simulink model "aerodynamic_tests"  (R2020a)
settings: Solver=FixedStepAuto  StartTime=0.0  StopTime=5  FixedStep=1e-5  RelTol=1e-3
undefined symbols (not defined in the file or in its folder): A4, AQ3483, AS4, BB3483
libraries: simulink x2, aerolibconvert2 x1
settings Model: SimulationMode=accelerator  Creator=rag  LastModifiedBy=rag

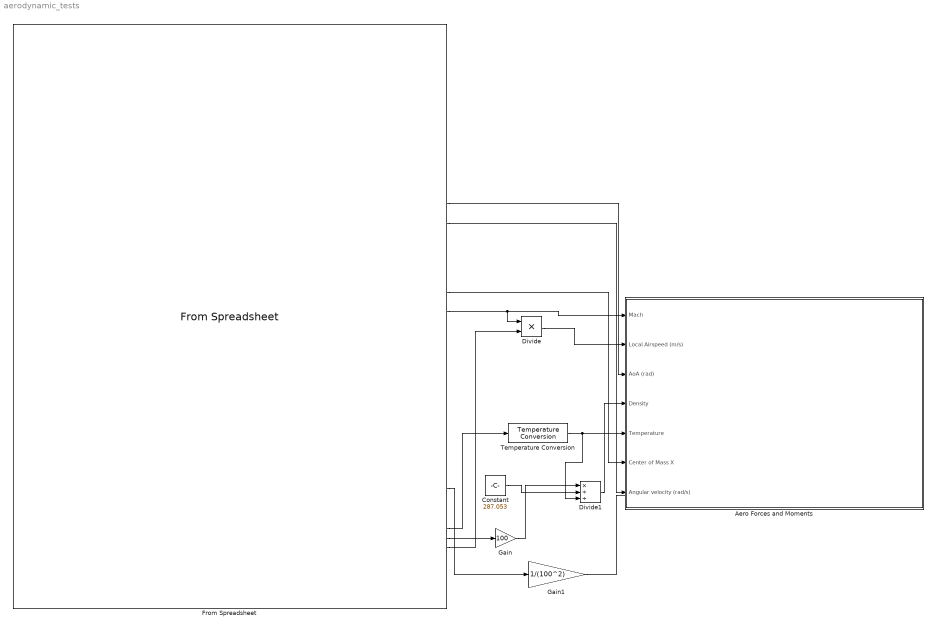
== system aerodynamic_tests ==
  Aero Forces and Moments : Subsystem
  Constant : Constant  Value=287.053
  Divide : Product  Inputs=**
  Divide1 : Product  Inputs=*//
  From Spreadsheet : FromSpreadsheet  FileName=C:\Users\rag\Documents\GitHub\EPQ\OpenRocket\full simulation F15 east 2.xlsx  SheetName=full simulation F15 east 2  Range=A4:AQ3483,AS4:BB3483  ExtrapolationBeforeFirstDataPoint=Hold first value  InterpolationWithinTimeRange=Zero order hold  ExtrapolationAfterLastDataPoint=Hold last value
  Gain : Gain  Gain=100
  Gain1 : Gain  Gain=1/(100^2)
  Temperature Conversion : aerolibconvert2/Temperature Conversion  IU=C  OU=K
      settings: SourceProductBaseCode=AE
  wires:
  From Spreadsheet/26 -> Divide/1, Aero Forces and Moments/1(Mach)
  From Spreadsheet/15 -> Aero Forces and Moments/3(AoA (rad))
  Divide1/1 -> Aero Forces and Moments/4(Density)
  From Spreadsheet/24 -> Aero Forces and Moments/6(Center of Mass X)
  From Spreadsheet/17 -> Aero Forces and Moments/7(Angular velocity (rad/s))
  Divide/1 -> Aero Forces and Moments/2(Local Airspeed (m/s))
  Temperature Conversion/1 -> Divide1/3, Aero Forces and Moments/5(Temperature)
  From Spreadsheet/48 -> Temperature Conversion/1
  From Spreadsheet/50 -> Divide/2
  Constant/1 -> Divide1/2
  From Spreadsheet/49 -> Gain/1
  Gain/1 -> Divide1/1
  Gain1/1 -> ?
  From Spreadsheet/44 -> Gain1/1

== system aerodynamic_tests/Aero Forces and Moments ==
  Mach : Inport
  Local Airspeed (m/s) : Inport  Port=2
  AoA (rad) : Inport  Port=3
  Density : Inport  Port=4
  Temperature : Inport  Port=5
  Center of Mass X : Inport  Port=6
  Angular velocity (rad/s) : Inport  Port=7
  Axial Drag Calculator : Subsystem
  CN and Cm calculator : Subsystem
  Constants : Subsystem
  wires:
  AoA (rad)/1 -> Axial Drag Calculator/2(AoA (rad)), CN and Cm calculator/3(AoA (rads))
  Temperature/1 -> Axial Drag Calculator/4(Temperature)
  Mach/1 -> CN and Cm calculator/1(Mach), Axial Drag Calculator/1(Mach)
  Density/1 -> Axial Drag Calculator/3(Density)
  Angular velocity (rad/s)/1 -> CN and Cm calculator/5(Angular Velocity (rad/s))
  Center of Mass X/1 -> CN and Cm calculator/4(Center of Mass X)
  Local Airspeed (m/s)/1 -> Axial Drag Calculator/13(Airspeed), CN and Cm calculator/2(Airspeed (m/s))
  Constants/1(Reference diameter (m)) -> CN and Cm calculator/7(Reference Diameter (m))
  Constants/3(Reference area (m^2)) -> Axial Drag Calculator/9(Reference Area (m^2)), CN and Cm calculator/8(Reference Area (m^2))
  Constants/4(Nose Cone Length (m)) -> Axial Drag Calculator/10(Nose Cone Length (m)), CN and Cm calculator/9(Nose Cone Length (m))
  Constants/5(Body Tube Length (m)) -> Axial Drag Calculator/5(Body Tube Length (m)), CN and Cm calculator/10(Body Tube Length (m))
  Constants/8(Nose Cone Planform Area (m^2)) -> CN and Cm calculator/11(Nose Cone Planform Area (m^2))
  Constants/9(Body Tube Planform Area (m^2)) -> CN and Cm calculator/12(Body Tube Planform Area (m^2))
  Constants/12(Body Tube CP (m)) -> CN and Cm calculator/13(Body Tube CP)
  Constants/13(Nose Cone CP (m)) -> CN and Cm calculator/14(Nose Cone CP)
  Constants/14(Pitch Center X (m)) -> CN and Cm calculator/15(Pitch Center X)
  Constants/7(Body Tube Wet Area (m^2)) -> Axial Drag Calculator/6(Body Tube Wet Area (m^2))
  Constants/6("Nose Cone Wet Area (m^2) ") -> Axial Drag Calculator/7(Nose Cone Wet Area (m^2))
  Constants/2(Reference radius (m)) -> Axial Drag Calculator/8(Reference Radius (m))
  Constants/10(Surface Roughness (m)) -> Axial Drag Calculator/11(Surface Roughness)
  Constants/11(sin(phi)) -> Axial Drag Calculator/12(sinphi)

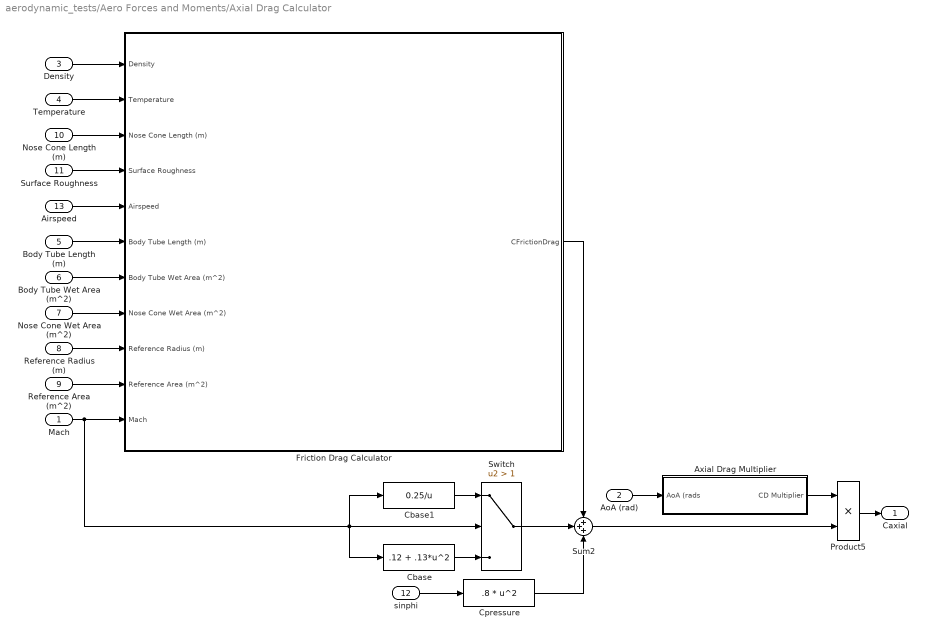
== system aerodynamic_tests/Aero Forces and Moments/Axial Drag Calculator ==
  Mach : Inport
  AoA (rad) : Inport  Port=2
  Density : Inport  Port=3
  Temperature : Inport  Port=4
  Body Tube Length (m) : Inport  Port=5
  Body Tube Wet Area (m^2) : Inport  Port=6
  Nose Cone Wet Area (m^2) : Inport  Port=7
  Reference Radius (m) : Inport  Port=8
  Reference Area (m^2) : Inport  Port=9
  Nose Cone Length (m) : Inport  Port=10
  Surface Roughness : Inport  Port=11
  sinphi : Inport  Port=12
  Airspeed : Inport  Port=13
  Axial Drag Multiplier : Subsystem
  Cbase : Fcn  Expr=.12 + .13*u^2
  Cbase1 : Fcn  Expr=0.25/u
  Cpressure : Fcn  Expr=.8 * u^2
  Friction Drag Calculator : Subsystem
  Product5 : Product
  Sum2 : Sum  Inputs=+++
  Switch : Switch  Criteria=u2 > Threshold  Threshold=1
  Caxial : Outport  VectorParamsAs1DForOutWhenUnconnected=off
  wires:
  Nose Cone Wet Area (m^2)/1 -> Friction Drag Calculator/8(Nose Cone Wet Area (m^2))
  Reference Area (m^2)/1 -> Friction Drag Calculator/10(Reference Area (m^2))
  Reference Radius (m)/1 -> Friction Drag Calculator/9(Reference Radius (m))
  Body Tube Wet Area (m^2)/1 -> Friction Drag Calculator/7(Body Tube Wet Area (m^2))
  sinphi/1 -> Cpressure/1
  Airspeed/1 -> Friction Drag Calculator/5(Airspeed)
  Surface Roughness/1 -> Friction Drag Calculator/4(Surface Roughness)
  Temperature/1 -> Friction Drag Calculator/2(Temperature)
  Mach/1 -> Cbase/1, Cbase1/1, Switch/2, Friction Drag Calculator/11(Mach)
  Density/1 -> Friction Drag Calculator/1(Density)
  Nose Cone Length (m)/1 -> Friction Drag Calculator/3(Nose Cone Length (m))
  Body Tube Length (m)/1 -> Friction Drag Calculator/6(Body Tube Length (m))
  Product5/1 -> Caxial/1
  Friction Drag Calculator/1(CFrictionDrag) -> Sum2/1
  Cbase/1 -> Switch/3
  Cpressure/1 -> Sum2/3
  AoA (rad)/1 -> Axial Drag Multiplier/1(AoA (rads)
  Sum2/1 -> Product5/2
  Axial Drag Multiplier/1(CD Multiplier) -> Product5/1
  Cbase1/1 -> Switch/1
  Switch/1 -> Sum2/2

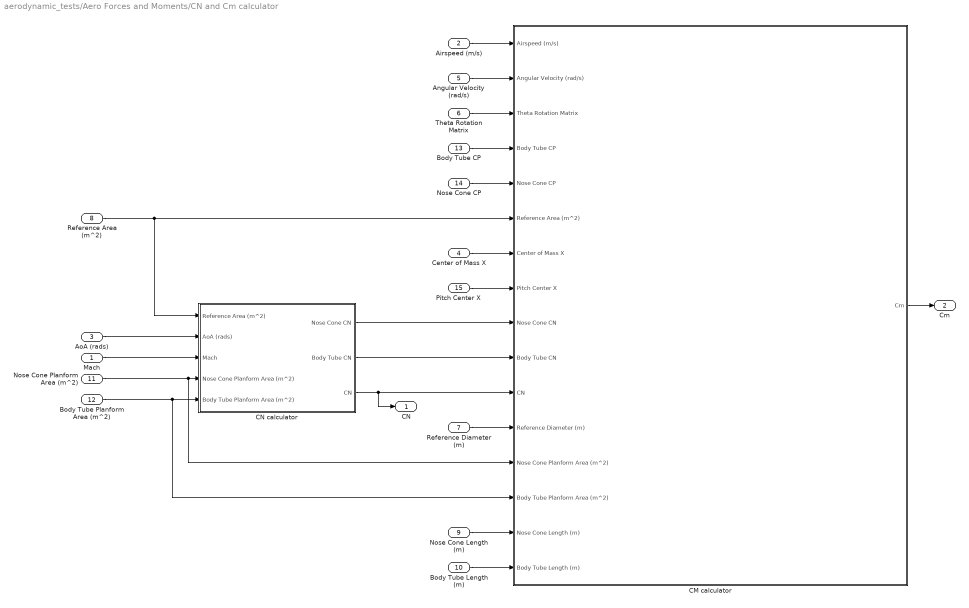
== system aerodynamic_tests/Aero Forces and Moments/CN and Cm calculator ==
  Mach : Inport
  Airspeed (m/s) : Inport  Port=2
  AoA (rads) : Inport  Port=3
  Center of Mass X : Inport  Port=4
  Angular Velocity (rad/s) : Inport  Port=5
  Theta Rotation Matrix : Inport  Port=6
  Reference Diameter (m) : Inport  Port=7
  Reference Area (m^2) : Inport  Port=8
  Nose Cone Length (m) : Inport  Port=9
  Body Tube Length (m) : Inport  Port=10
  Nose Cone Planform Area (m^2) : Inport  Port=11
  Body Tube Planform Area (m^2) : Inport  Port=12
  Body Tube CP : Inport  Port=13
  Nose Cone CP : Inport  Port=14
  Pitch Center X : Inport  Port=15
  CM calculator : Subsystem
  CN calculator : Subsystem
  CN : Outport  VectorParamsAs1DForOutWhenUnconnected=off
  Cm : Outport  Port=2  VectorParamsAs1DForOutWhenUnconnected=off
  wires:
  Body Tube Planform Area (m^2)/1 -> CM calculator/14(Body Tube Planform Area (m^2)), CN calculator/5(Body Tube Planform Area (m^2))
  Pitch Center X/1 -> CM calculator/8(Pitch Center X)
  Nose Cone CP/1 -> CM calculator/5(Nose Cone CP)
  Body Tube CP/1 -> CM calculator/4(Body Tube CP)
  Nose Cone Planform Area (m^2)/1 -> CM calculator/13(Nose Cone Planform Area (m^2)), CN calculator/4(Nose Cone Planform Area (m^2))
  Angular Velocity (rad/s)/1 -> CM calculator/2(Angular Velocity (rad/s))
  Reference Area (m^2)/1 -> CN calculator/1(Reference Area (m^2)), CM calculator/6(Reference Area (m^2))
  AoA (rads)/1 -> CN calculator/2(AoA (rads))
  Mach/1 -> CN calculator/3(Mach)
  Center of Mass X/1 -> CM calculator/7(Center of Mass X)
  CN calculator/3(CN) -> CN/1, CM calculator/11(CN)
  CN calculator/2(Body Tube CN) -> CM calculator/10(Body Tube CN)
  CN calculator/1(Nose Cone CN) -> CM calculator/9(Nose Cone CN)
  Airspeed (m/s)/1 -> CM calculator/1(Airspeed (m/s))
  Theta Rotation Matrix/1 -> CM calculator/3(Theta Rotation Matrix)
  Reference Diameter (m)/1 -> CM calculator/12(Reference Diameter (m))
  Nose Cone Length (m)/1 -> CM calculator/15(Nose Cone Length (m))
  CM calculator/1(Cm) -> Cm/1
  Body Tube Length (m)/1 -> CM calculator/16(Body Tube Length (m))

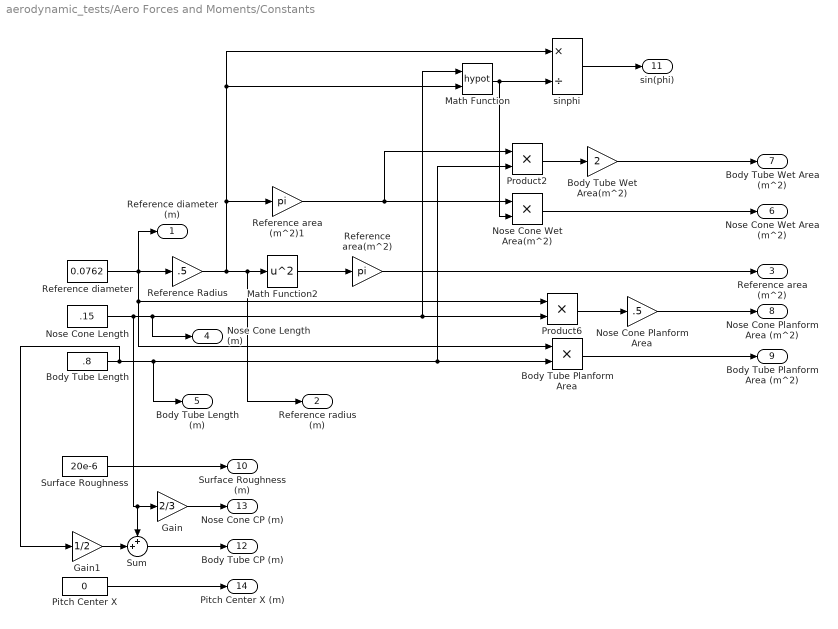
== system aerodynamic_tests/Aero Forces and Moments/Constants ==
  Body Tube Length : Constant  Value=.8
  Body Tube Planform Area : Product
  Body Tube Wet Area(m^2) : Gain  Gain=2
  Gain : Gain  Gain=2/3
  Gain1 : Gain  Gain=1/2
  Math Function : Math  Operator=hypot  SignedPower=on  SaturateOnIntegerOverflow=on
  Math Function2 : Math  Operator=square  SignedPower=on  SaturateOnIntegerOverflow=on
  Nose Cone Length : Constant  Value=.15
  Nose Cone Planform Area : Gain  Gain=.5
  Nose Cone Wet Area(m^2) : Product
  Pitch Center X : Constant  Value=0
  Product2 : Product
  Product6 : Product
  Reference Radius : Gain  Gain=.5
  Reference area (m^2)1 : Gain  Gain=pi
  Reference area(m^2) : Gain  Gain=pi
  Reference diameter : Constant  Value=0.0762
  Sum : Sum  Inputs=++|
  Surface Roughness : Constant  Value=20e-6
  sinphi : Product  Inputs=*/
  Reference diameter (m) : Outport  VectorParamsAs1DForOutWhenUnconnected=off
  Reference radius (m) : Outport  Port=2  VectorParamsAs1DForOutWhenUnconnected=off
  Reference area (m^2) : Outport  Port=3  VectorParamsAs1DForOutWhenUnconnected=off
  Nose Cone Length (m) : Outport  Port=4  VectorParamsAs1DForOutWhenUnconnected=off
  Body Tube Length (m) : Outport  Port=5  VectorParamsAs1DForOutWhenUnconnected=off
  "Nose Cone Wet Area (m^2) " : Outport  Port=6  VectorParamsAs1DForOutWhenUnconnected=off
  Body Tube Wet Area (m^2) : Outport  Port=7  VectorParamsAs1DForOutWhenUnconnected=off
  Nose Cone Planform Area (m^2) : Outport  Port=8  VectorParamsAs1DForOutWhenUnconnected=off
  Body Tube Planform Area (m^2) : Outport  Port=9  VectorParamsAs1DForOutWhenUnconnected=off
  Surface Roughness (m) : Outport  Port=10  VectorParamsAs1DForOutWhenUnconnected=off
  sin(phi) : Outport  Port=11  VectorParamsAs1DForOutWhenUnconnected=off
  Body Tube CP (m) : Outport  Port=12  VectorParamsAs1DForOutWhenUnconnected=off
  Nose Cone CP (m) : Outport  Port=13  VectorParamsAs1DForOutWhenUnconnected=off
  Pitch Center X (m) : Outport  Port=14  VectorParamsAs1DForOutWhenUnconnected=off
  wires:
  Reference diameter/1 -> Reference diameter (m)/1, Body Tube Planform Area/1, Product6/1, Reference Radius/1
  Math Function2/1 -> Reference area(m^2)/1
  Nose Cone Length/1 -> Product6/2, Math Function/1, Nose Cone Length (m)/1, Sum/1, Gain/1
  Product6/1 -> Nose Cone Planform Area/1
  Reference Radius/1 -> Math Function2/1, Reference radius (m)/1, Math Function/2, sinphi/1, Reference area (m^2)1/1
  Reference area (m^2)1/1 -> Product2/1, Nose Cone Wet Area(m^2)/1
  Product2/1 -> Body Tube Wet Area(m^2)/1
  Math Function/1 -> Nose Cone Wet Area(m^2)/2, sinphi/2
  Reference area(m^2)/1 -> Reference area (m^2)/1
  Nose Cone Wet Area(m^2)/1 -> "Nose Cone Wet Area (m^2) "/1
  Body Tube Wet Area(m^2)/1 -> Body Tube Wet Area (m^2)/1
  Body Tube Planform Area/1 -> Body Tube Planform Area (m^2)/1
  Nose Cone Planform Area/1 -> Nose Cone Planform Area (m^2)/1
  Surface Roughness/1 -> Surface Roughness (m)/1
  sinphi/1 -> sin(phi)/1
  Sum/1 -> Body Tube CP (m)/1
  Gain/1 -> Nose Cone CP (m)/1
  Pitch Center X/1 -> Pitch Center X (m)/1
  Gain1/1 -> Sum/2
  Body Tube Length/1 -> Gain1/1, Body Tube Length (m)/1, Body Tube Planform Area/2, Product2/2

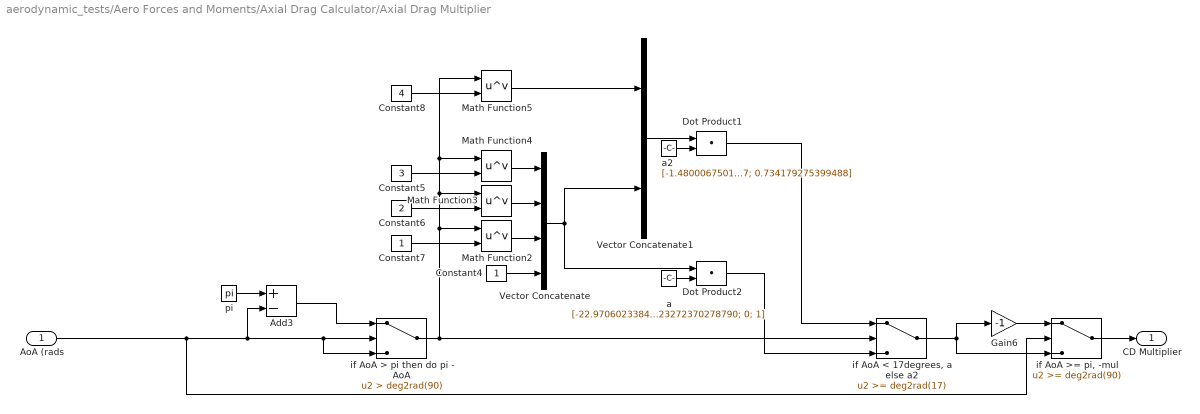
== system aerodynamic_tests/Aero Forces and Moments/Axial Drag Calculator/Axial Drag Multiplier ==
  AoA (rads : Inport
  Add3 : Sum  Inputs=+-
  Constant4 : Constant
  Constant5 : Constant  Value=3
  Constant6 : Constant  Value=2
  Constant7 : Constant
  Constant8 : Constant  Value=4
  Dot Product1 : DotProduct  SaturateOnIntegerOverflow=on  OutDataTypeStr=Inherit: Inherit via internal rule
  Dot Product2 : DotProduct  SaturateOnIntegerOverflow=on  OutDataTypeStr=Inherit: Inherit via internal rule
  Gain6 : Gain  Gain=-1
  Math Function{2..5} (4 alike) : Math  Operator=pow  SignedPower=on  SaturateOnIntegerOverflow=on
  Vector Concatenate : Concatenate  NumInputs=4
  Vector Concatenate1 : Concatenate
  a : Constant  Value=[-22.970602338418825; 10.223272370278790; 0; 1]
  a2 : Constant  Value=[-1.480006750190687; 6.784940235048046; -10.062655893223173; 4.334008218595027; 0.734179275399488]
  "if AoA < 17degrees, a else a2" : Switch  Threshold=deg2rad(17)
  if AoA > pi then do pi - AoA : Switch  Criteria=u2 > Threshold  Threshold=deg2rad(90)
  "if AoA >= pi, -mul" : Switch  Threshold=deg2rad(90)
  pi : Constant  Value=pi
  CD Multiplier : Outport  VectorParamsAs1DForOutWhenUnconnected=off
  wires:
  Constant4/1 -> Vector Concatenate/4
  Constant5/1 -> Math Function4/2
  if AoA > pi then do pi - AoA/1 -> Math Function5/1, Math Function4/1, Math Function3/1, Math Function2/1, "if AoA < 17degrees, a else a2"/2
  Add3/1 -> if AoA > pi then do pi - AoA/1
  Vector Concatenate1/1 -> Dot Product1/1
  AoA (rads/1 -> "if AoA >= pi, -mul"/2, Add3/2, if AoA > pi then do pi - AoA/3, if AoA > pi then do pi - AoA/2
  a/1 -> Dot Product2/2
  "if AoA >= pi, -mul"/1 -> CD Multiplier/1
  Math Function4/1 -> Vector Concatenate/1
  "if AoA < 17degrees, a else a2"/1 -> "if AoA >= pi, -mul"/3, Gain6/1
  Gain6/1 -> "if AoA >= pi, -mul"/1
  pi/1 -> Add3/1
  Constant7/1 -> Math Function2/2
  Vector Concatenate/1 -> Vector Concatenate1/2, Dot Product2/1
  Math Function2/1 -> Vector Concatenate/3
  Constant6/1 -> Math Function3/2
  Dot Product2/1 -> "if AoA < 17degrees, a else a2"/3
  Constant8/1 -> Math Function5/2
  a2/1 -> Dot Product1/2
  Math Function5/1 -> Vector Concatenate1/1
  Math Function3/1 -> Vector Concatenate/2
  Dot Product1/1 -> "if AoA < 17degrees, a else a2"/1

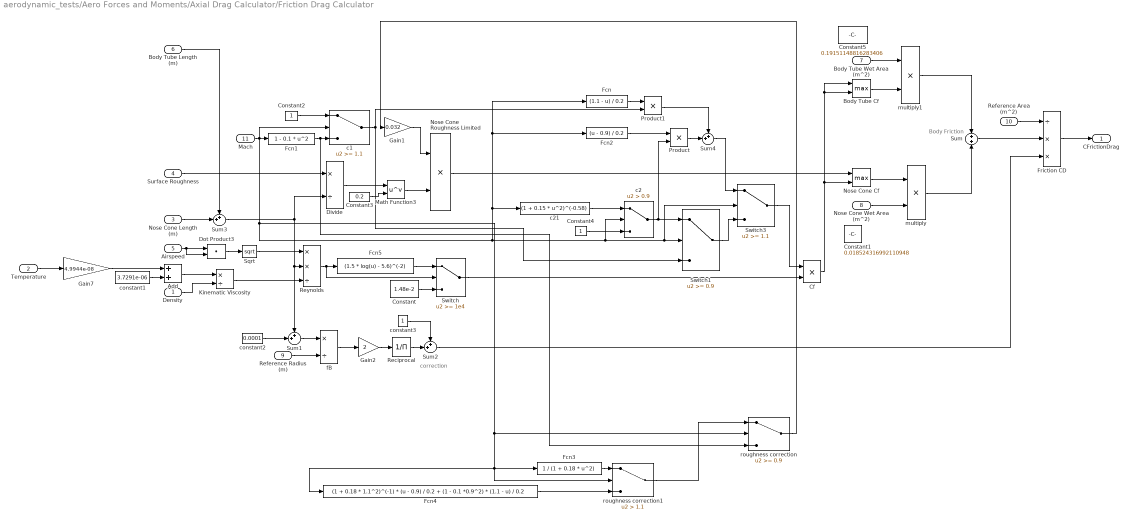
== system aerodynamic_tests/Aero Forces and Moments/Axial Drag Calculator/Friction Drag Calculator ==
  note: correction
  note: Body Friction
  Density : Inport
  Temperature : Inport  Port=2
  Nose Cone Length (m) : Inport  Port=3
  Surface Roughness : Inport  Port=4
  Airspeed : Inport  Port=5
  Body Tube Length (m) : Inport  Port=6
  Body Tube Wet Area (m^2) : Inport  Port=7
  Nose Cone Wet Area (m^2) : Inport  Port=8
  Reference Radius (m) : Inport  Port=9
  Reference Area (m^2) : Inport  Port=10
  Mach : Inport  Port=11
  Add : Sum
  Body Tube Cf : MinMax  Function=max  Inputs=2
  Cf : Product  Inputs=**
  Constant : Constant  Value=1.48e-2
  Constant1 : Constant  Value=0.018524316992110948
  Constant2 : Constant
  Constant3 : Constant  Value=0.2
  Constant4 : Constant
  Constant5 : Constant  Value=0.19151148816283406
  Divide : Product  Inputs=*/
  Dot Product3 : DotProduct  SaturateOnIntegerOverflow=on  OutDataTypeStr=Inherit: Inherit via internal rule
  Fcn : Fcn  Expr=(1.1 - u) / 0.2
  Fcn1 : Fcn  Expr=1 - 0.1 * u^2
  Fcn2 : Fcn  Expr=(u - 0.9) / 0.2
  Fcn3 : Fcn  Expr=1 / (1 + 0.18 * u^2)
  Fcn4 : Fcn  Expr=(1 + 0.18 * 1.1^2)^(-1) * (u - 0.9) / 0.2 + (1 - 0.1 *0.9^2) * (1.1 - u) / 0.2
  Fcn5 : Fcn  Expr=(1.5 * log(u) - 5.6)^(-2)
  Friction CD : Product  Inputs=/**
  Gain1 : Gain  Gain=0.032
  Gain2 : Gain  Gain=2
  Gain7 : Gain  Gain=4.9944e-08
  Kinematic Viscosity : Product  Inputs=*/
  Math Function3 : Math  Operator=pow  SignedPower=on  SaturateOnIntegerOverflow=on
  Nose Cone Cf : MinMax  Function=max  Inputs=2
  Nose Cone Roughness Limited : Product  Inputs=**
  Product : Product
  Product1 : Product
  Reciprocal : Product  Inputs=/
  Reynolds : Product  Inputs=**/
  Sqrt : Sqrt  SaturateOnIntegerOverflow=on
  Sum : Sum
  Sum{1..4} (4 alike) : Sum  Inputs=++|
  Switch : Switch  Threshold=1e4
  Switch1 : Switch  Threshold=0.9
  Switch3 : Switch  Threshold=1.1
  c1 : Switch  Threshold=1.1
  c2 : Switch  Criteria=u2 > Threshold  Threshold=0.9
  c21 : Fcn  Expr=(1 + 0.15 * u^2)^(-0.58)
  constant1 : Constant  Value=3.7291e-06
  constant2 : Constant  Value=0.0001
  constant3 : Constant
  fB : Product  Inputs=*/
  multiply : Product  Inputs=**
  multiply1 : Product  Inputs=**
  roughness correction : Switch  Threshold=0.9
  roughness correction1 : Switch  Criteria=u2 > Threshold  Threshold=1.1
  CFrictionDrag : Outport  VectorParamsAs1DForOutWhenUnconnected=off
  wires:
  Sqrt/1 -> Reynolds/1
  Kinematic Viscosity/1 -> Reynolds/3
  Constant3/1 -> Math Function3/2
  constant1/1 -> Add/2
  Add/1 -> Kinematic Viscosity/1
  Gain7/1 -> Add/1
  Reynolds/1 -> Switch/2, Fcn5/1
  Gain1/1 -> Nose Cone Roughness Limited/1
  Divide/1 -> Math Function3/1
  Math Function3/1 -> Nose Cone Roughness Limited/2
  Surface Roughness/1 -> Divide/1
  Temperature/1 -> Gain7/1
  Density/1 -> Kinematic Viscosity/2
  Nose Cone Roughness Limited/1 -> Nose Cone Cf/1
  Nose Cone Length (m)/1 -> Sum3/2
  Body Tube Length (m)/1 -> Sum3/1
  Cf/1 -> Body Tube Cf/1, Body Tube Cf/2, Nose Cone Cf/2
  Nose Cone Cf/1 -> multiply/1
  Nose Cone Wet Area (m^2)/1 -> multiply/2
  Body Tube Wet Area (m^2)/1 -> multiply1/1
  Body Tube Cf/1 -> multiply1/2
  multiply/1 -> Sum/2
  multiply1/1 -> Sum/1
  constant2/1 -> Sum1/2
  Sum1/1 -> fB/1
  Reference Radius (m)/1 -> fB/2
  fB/1 -> Gain2/1
  Gain2/1 -> Reciprocal/1
  Reciprocal/1 -> Sum2/2
  constant3/1 -> Sum2/1
  Sum/1 -> Friction CD/2
  Sum2/1 -> Friction CD/3
  Reference Area (m^2)/1 -> Friction CD/1
  Friction CD/1 -> CFrictionDrag/1
  Airspeed/1 -> Dot Product3/2, Dot Product3/1
  Dot Product3/1 -> Sqrt/1
  Switch/1 -> Cf/2
  Fcn5/1 -> Switch/1
  Constant/1 -> Switch/3
  c1/1 -> Product1/2, Switch1/3
  Fcn1/1 -> roughness correction/3, c1/3
  Constant2/1 -> c1/1
  c2/1 -> Product/2, Switch1/1
  Constant4/1 -> c2/3
  c21/1 -> c2/1
  Switch3/1 -> Cf/1
  Switch1/1 -> Switch3/3
  Fcn2/1 -> Product/1
  Product/1 -> Sum4/2
  Product1/1 -> Sum4/1
  Fcn/1 -> Product1/1
  Sum4/1 -> Switch3/1
  Fcn3/1 -> roughness correction1/1
  Mach/1 -> roughness correction/2, Fcn4/1, roughness correction1/2, Fcn3/1, Fcn/1, Fcn2/1, c21/1, c2/2, Switch3/2, Switch1/2, c1/2, Fcn1/1
  Fcn4/1 -> roughness correction1/3
  roughness correction1/1 -> roughness correction/1
  roughness correction/1 -> Gain1/1
  Sum3/1 -> Divide/2, Sum1/1, Reynolds/2

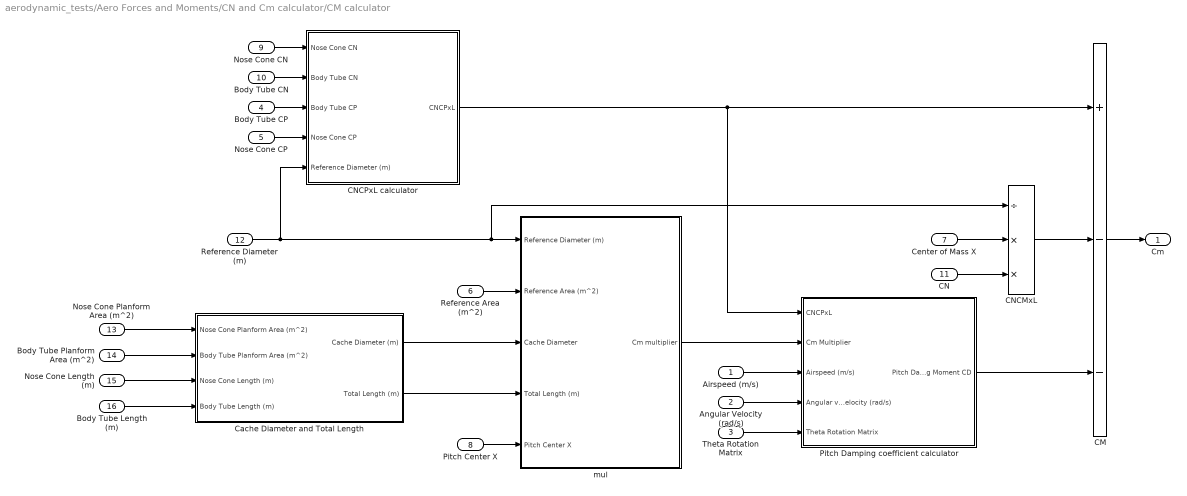
== system aerodynamic_tests/Aero Forces and Moments/CN and Cm calculator/CM calculator ==
  Airspeed (m/s) : Inport
  Angular Velocity (rad/s) : Inport  Port=2
  Theta Rotation Matrix : Inport  Port=3
  Body Tube CP : Inport  Port=4
  Nose Cone CP : Inport  Port=5
  Reference Area (m^2) : Inport  Port=6
  Center of Mass X : Inport  Port=7
  Pitch Center X : Inport  Port=8
  Nose Cone CN : Inport  Port=9
  Body Tube CN : Inport  Port=10
  CN : Inport  Port=11
  Reference Diameter (m) : Inport  Port=12
  Nose Cone Planform Area (m^2) : Inport  Port=13
  Body Tube Planform Area (m^2) : Inport  Port=14
  Nose Cone Length (m) : Inport  Port=15
  Body Tube Length (m) : Inport  Port=16
  CM : Sum  Inputs=+--
  CNCMxL : Product  Inputs=/**
  CNCPxL calculator : Subsystem
  Cache Diameter and Total Length : Subsystem
  Pitch Damping coefficient calculator : Subsystem
  mul : Subsystem
  Cm : Outport  VectorParamsAs1DForOutWhenUnconnected=off
  wires:
  CNCPxL calculator/1("CNCPxL ") -> Pitch Damping coefficient calculator/1(CNCPxL), CM/1
  Pitch Center X/1 -> mul/5(Pitch Center X)
  Cache Diameter and Total Length/2(Total Length (m)) -> mul/4(Total Length (m))
  Reference Diameter (m)/1 -> CNCMxL/1, mul/1(Reference Diameter (m)), CNCPxL calculator/5(Reference Diameter (m))
  Nose Cone CP/1 -> CNCPxL calculator/4(Nose Cone CP)
  CM/1 -> Cm/1
  Body Tube CP/1 -> CNCPxL calculator/3(Body Tube CP)
  Cache Diameter and Total Length/1(Cache Diameter (m)) -> mul/3(Cache Diameter)
  mul/1(Cm multiplier) -> Pitch Damping coefficient calculator/2(Cm Multiplier)
  Angular Velocity (rad/s)/1 -> Pitch Damping coefficient calculator/4(Angular velocity (rad/s))
  Airspeed (m/s)/1 -> Pitch Damping coefficient calculator/3(Airspeed (m/s))
  Reference Area (m^2)/1 -> mul/2(Reference Area (m^2))
  Theta Rotation Matrix/1 -> Pitch Damping coefficient calculator/5(Theta Rotation Matrix)
  Body Tube CN/1 -> CNCPxL calculator/2(Body Tube CN)
  Nose Cone CN/1 -> CNCPxL calculator/1(Nose Cone CN)
  Nose Cone Planform Area (m^2)/1 -> Cache Diameter and Total Length/1(Nose Cone Planform Area (m^2))
  Body Tube Planform Area (m^2)/1 -> Cache Diameter and Total Length/2(Body Tube Planform Area (m^2))
  Nose Cone Length (m)/1 -> Cache Diameter and Total Length/3(Nose Cone Length (m))
  Body Tube Length (m)/1 -> Cache Diameter and Total Length/4(Body Tube Length (m))
  Center of Mass X/1 -> CNCMxL/2
  CN/1 -> CNCMxL/3
  Pitch Damping coefficient calculator/1(Pitch Damping Moment CD) -> CM/3
  CNCMxL/1 -> CM/2

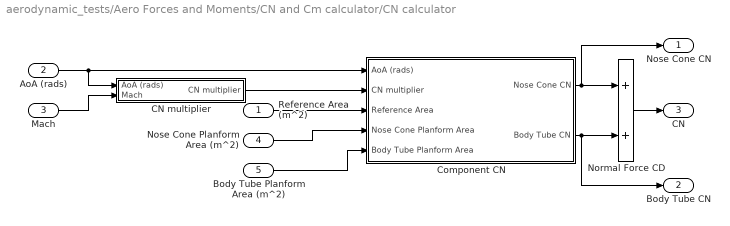
== system aerodynamic_tests/Aero Forces and Moments/CN and Cm calculator/CN calculator ==
  Reference Area (m^2) : Inport
  AoA (rads) : Inport  Port=2
  Mach : Inport  Port=3
  Nose Cone Planform Area (m^2) : Inport  Port=4
  Body Tube Planform Area (m^2) : Inport  Port=5
  CN multiplier : Subsystem
  Component CN : Subsystem
  Normal Force CD : Sum
  Nose Cone CN : Outport  VectorParamsAs1DForOutWhenUnconnected=off
  Body Tube CN : Outport  Port=2  VectorParamsAs1DForOutWhenUnconnected=off
  CN : Outport  Port=3  VectorParamsAs1DForOutWhenUnconnected=off
  wires:
  Mach/1 -> CN multiplier/2(Mach)
  CN multiplier/1(CN multiplier) -> Component CN/2(CN multiplier)
  Component CN/1(Nose Cone CN) -> Normal Force CD/1, Nose Cone CN/1
  AoA (rads)/1 -> CN multiplier/1(AoA (rads)), Component CN/1(AoA (rads))
  Nose Cone Planform Area (m^2)/1 -> Component CN/4(Nose Cone Planform Area)
  Component CN/2(Body Tube CN) -> Normal Force CD/2, Body Tube CN/1
  Body Tube Planform Area (m^2)/1 -> Component CN/5(Body Tube Planform Area)
  Reference Area (m^2)/1 -> Component CN/3(Reference Area)
  Normal Force CD/1 -> CN/1

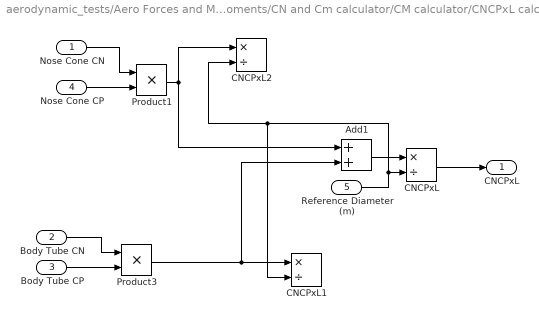
== system aerodynamic_tests/Aero Forces and Moments/CN and Cm calculator/CM calculator/CNCPxL calculator ==
  Nose Cone CN : Inport
  Body Tube CN : Inport  Port=2
  Body Tube CP : Inport  Port=3
  Nose Cone CP : Inport  Port=4
  Reference Diameter (m) : Inport  Port=5
  Add1 : Sum
  CNCPxL : Product  Inputs=*/
  CNCPxL1 : Product  Inputs=*/
  CNCPxL2 : Product  Inputs=*/
  Product1 : Product
  Product3 : Product
  "CNCPxL " : Outport  VectorParamsAs1DForOutWhenUnconnected=off
  wires:
  Product1/1 -> Add1/1, CNCPxL2/1
  CNCPxL/1 -> "CNCPxL "/1
  Nose Cone CN/1 -> Product1/1
  Reference Diameter (m)/1 -> CNCPxL2/2, CNCPxL1/2, CNCPxL/2
  Body Tube CN/1 -> Product3/1
  Add1/1 -> CNCPxL/1
  Body Tube CP/1 -> Product3/2
  Product3/1 -> CNCPxL1/1, Add1/2
  Nose Cone CP/1 -> Product1/2

== system aerodynamic_tests/Aero Forces and Moments/CN and Cm calculator/CM calculator/Cache Diameter and Total Length ==
  Nose Cone Planform Area (m^2) : Inport
  Body Tube Planform Area (m^2) : Inport  Port=2
  Nose Cone Length (m) : Inport  Port=3
  Body Tube Length (m) : Inport  Port=4
  Cache Diameter : Product  Inputs=*/
  Total Length : Sum
  Total Planform Area : Sum
  Cache Diameter (m) : Outport  VectorParamsAs1DForOutWhenUnconnected=off
  Total Length (m) : Outport  Port=2  VectorParamsAs1DForOutWhenUnconnected=off
  wires:
  Total Planform Area/1 -> Cache Diameter/1
  Nose Cone Planform Area (m^2)/1 -> Total Planform Area/1
  Body Tube Length (m)/1 -> Total Length/2
  Nose Cone Length (m)/1 -> Total Length/1
  Body Tube Planform Area (m^2)/1 -> Total Planform Area/2
  Total Length/1 -> Total Length (m)/1, Cache Diameter/2
  Cache Diameter/1 -> Cache Diameter (m)/1

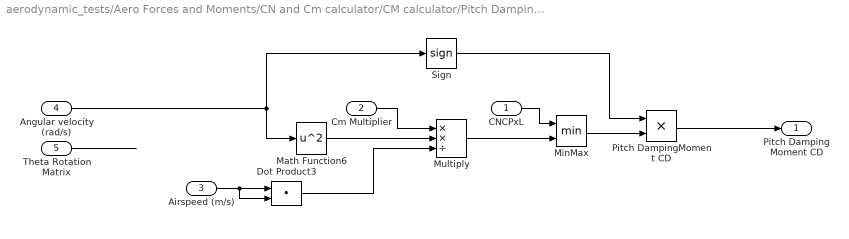
== system aerodynamic_tests/Aero Forces and Moments/CN and Cm calculator/CM calculator/Pitch Damping coefficient calculator ==
  CNCPxL : Inport
  Cm Multiplier : Inport  Port=2
  Airspeed (m/s) : Inport  Port=3
  Angular velocity (rad/s) : Inport  Port=4
  Theta Rotation Matrix : Inport  Port=5
  Dot Product3 : DotProduct  SaturateOnIntegerOverflow=on  OutDataTypeStr=Inherit: Inherit via internal rule
  Math Function6 : Math  Operator=square  SignedPower=on  SaturateOnIntegerOverflow=on
  MinMax : MinMax  Inputs=2
  Multiply : Product  Inputs=**/
  Pitch DampingMoment CD : Product
  Sign : Signum
  Pitch Damping Moment CD : Outport  VectorParamsAs1DForOutWhenUnconnected=off
  wires:
  Dot Product3/1 -> Multiply/3
  Airspeed (m/s)/1 -> Dot Product3/2, Dot Product3/1
  Sign/1 -> Pitch DampingMoment CD/1
  CNCPxL/1 -> MinMax/1
  Math Function6/1 -> Multiply/2
  Multiply/1 -> MinMax/2
  Pitch DampingMoment CD/1 -> Pitch Damping Moment CD/1
  Angular velocity (rad/s)/1 -> Math Function6/1, Sign/1
  MinMax/1 -> Pitch DampingMoment CD/2
  Theta Rotation Matrix/1 -> ?
  Cm Multiplier/1 -> Multiply/1

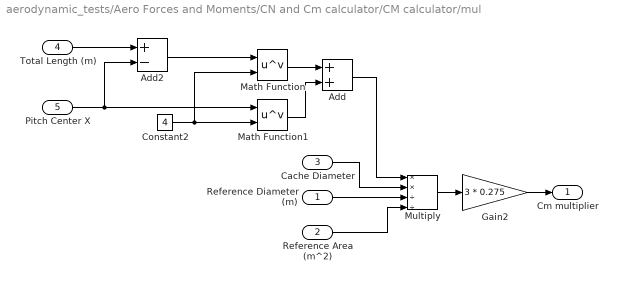
== system aerodynamic_tests/Aero Forces and Moments/CN and Cm calculator/CM calculator/mul ==
  Reference Diameter (m) : Inport
  Reference Area (m^2) : Inport  Port=2
  Cache Diameter : Inport  Port=3
  Total Length (m) : Inport  Port=4
  Pitch Center X : Inport  Port=5
  Add : Sum
  Add2 : Sum  Inputs=+-
  Constant2 : Constant  Value=4
  Gain2 : Gain  Gain=3 * 0.275
  Math Function : Math  Operator=pow  SignedPower=on  SaturateOnIntegerOverflow=on
  Math Function1 : Math  Operator=pow  SignedPower=on  SaturateOnIntegerOverflow=on
  Multiply : Product  Inputs=**//
  Cm multiplier : Outport  VectorParamsAs1DForOutWhenUnconnected=off
  wires:
  Math Function1/1 -> Add/2
  Pitch Center X/1 -> Add2/2, Math Function1/1
  Constant2/1 -> Math Function/2, Math Function1/2
  Add/1 -> Multiply/1
  Math Function/1 -> Add/1
  Reference Area (m^2)/1 -> Multiply/4
  Multiply/1 -> Gain2/1
  Add2/1 -> Math Function/1
  Reference Diameter (m)/1 -> Multiply/3
  Gain2/1 -> Cm multiplier/1
  Total Length (m)/1 -> Add2/1
  Cache Diameter/1 -> Multiply/2

== system aerodynamic_tests/Aero Forces and Moments/CN and Cm calculator/CN calculator/CN multiplier ==
  AoA (rads) : Inport
  Mach : Inport  Port=2
  1 : Constant
  Compare To Constant : simulink/Logic and Bit Operations/Compare To Constant  relop=<  const=.05  OutDataTypeStr=boolean
  Compare To Constant1 : simulink/Logic and Bit Operations/Compare To Constant  relop=>  const=pi/4  OutDataTypeStr=boolean
  Gain : Gain  Gain=1/0.05
  Logical Operator : Logic  AllPortsSameDT=off  OutDataTypeStr=boolean
  Square : Math  Operator=square  SignedPower=on  SaturateOnIntegerOverflow=on
  cnmul : Switch  Criteria=u2 > Threshold
  CN multiplier : Outport  VectorParamsAs1DForOutWhenUnconnected=off
  wires:
  AoA (rads)/1 -> Compare To Constant1/1
  Logical Operator/1 -> cnmul/2
  Compare To Constant/1 -> Logical Operator/2
  Mach/1 -> Compare To Constant/1, Gain/1
  Compare To Constant1/1 -> Logical Operator/1
  Square/1 -> cnmul/1
  1/1 -> cnmul/3
  Gain/1 -> Square/1
  cnmul/1 -> CN multiplier/1

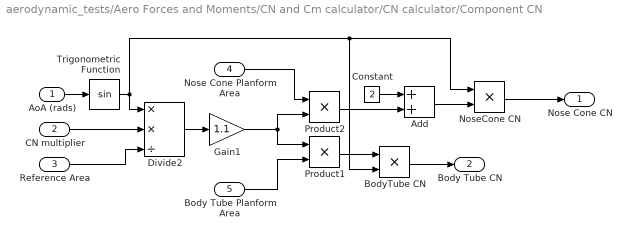
== system aerodynamic_tests/Aero Forces and Moments/CN and Cm calculator/CN calculator/Component CN ==
  AoA (rads) : Inport
  CN multiplier : Inport  Port=2
  Reference Area : Inport  Port=3
  Nose Cone Planform Area : Inport  Port=4
  Body Tube Planform Area : Inport  Port=5
  Add : Sum
  BodyTube CN : Product
  Constant : Constant  Value=2
  Divide2 : Product  Inputs=**/
  Gain1 : Gain  Gain=1.1
  NoseCone CN : Product
  Product1 : Product
  Product2 : Product
  Trigonometric Function : Trigonometry
  Nose Cone CN : Outport  VectorParamsAs1DForOutWhenUnconnected=off
  Body Tube CN : Outport  Port=2  VectorParamsAs1DForOutWhenUnconnected=off
  wires:
  Body Tube Planform Area/1 -> Product1/2
  NoseCone CN/1 -> Nose Cone CN/1
  Constant/1 -> Add/1
  Nose Cone Planform Area/1 -> Product2/1
  Add/1 -> NoseCone CN/2
  BodyTube CN/1 -> Body Tube CN/1
  CN multiplier/1 -> Divide2/2
  AoA (rads)/1 -> Trigonometric Function/1
  Divide2/1 -> Gain1/1
  Reference Area/1 -> Divide2/3
  Gain1/1 -> Product2/2, Product1/1
  Product2/1 -> Add/2
  Trigonometric Function/1 -> Divide2/1, BodyTube CN/2, NoseCone CN/1
  Product1/1 -> BodyTube CN/1
